simulink model "HSV"  (R2016a)
settings: Solver=VariableStepAuto  StartTime=0.0  StopTime=10.0  RelTol=1e-3
values from neighbouring files (symbols this model uses):
  arc = pi/180.    (= 0.0174532925199)    [HSV6DOF.m]    (also in Simulink_Constants.m; aerodynamics.m; initiala.m)
  bref = 24.38/2    (= 12.19)    [Simulink_Constants.m]
  CD = interp1(alX,CDX,algr,'cubic')    [aerodynamics.m]
  chi0 = -0.01    [Simulink_Constants.m]
  CL = interp1(alX,CLX,algr,'cubic')*mue    [aerodynamics.m]
  Cm = interp1(alX,CmX,algr,'cubic')    [aerodynamics.m]
  Cn = interp1(b1X,CnX,begr,'cubic')    [aerodynamics.m]
  g0 = 9.806    [Simulink_Constants.m]
  gamma0 = -0.01    [Simulink_Constants.m]
  h_theta_phi0 = [30000 55*arc 37*arc]'    [Simulink_Constants.m]
  Ix = 1572748.82    [Simulink_Constants.m]
  Ixz = 379629.026    [Simulink_Constants.m]
  Iy = 31590558.23    [Simulink_Constants.m]
  Iz = 32539630.8    [Simulink_Constants.m]
  Lref = 22.86    [Simulink_Constants.m]    (also in constants.m = 8.4088)
  m = 9300    [constants.m]
  mass_0 = 136077.7    [Simulink_Constants.m]
  mass_e = 5.4431e+04    (= 54431)    [Simulink_Constants.m]
  mass_f = 136077.7    [Simulink_Constants.m]
  phi_theta_psi_0 = [0 0 0]'    [Simulink_Constants.m]
  pqrt_0 = [0 0 0]'    [Simulink_Constants.m]
  Rearth = 6.38E6    (= 6380000)    [Simulink_Constants.m]
  rho30000m = 0.1841    [Simulink_Constants.m]
  Sref = 557.42    [Simulink_Constants.m]    (also in constants.m = 21.672)
  Ub_Vb_Qb0 = [1830 0 0]'    [Simulink_Constants.m]
  xme_0 = [0 0 0]'    [Simulink_Constants.m]
undefined symbols (not defined in the file or in its folder): Cl, Cy, Isp, magnitude, s, Thrust
libraries: aerolibutil x5, aerolibtransform2 x1, aerolibbdyn x1, aerolibconvert2 x1, aerolib6dof2 x1, aerolibanim x1, aerolibasang x1
settings Model: Creator=Bakry  LastModifiedBy=Bakry

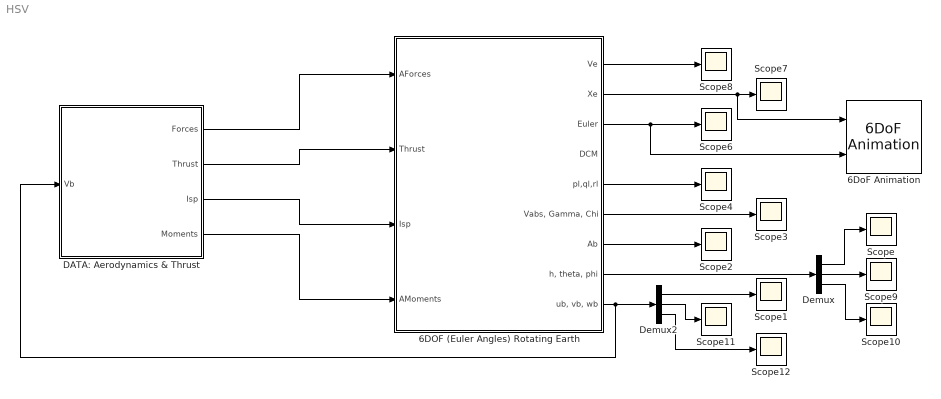
== system HSV ==
  6DOF (Euler Angles) Rotating Earth : Subsystem
  6DoF Animation : aerolibanim/6DoF Animation  u1=[0 4000 -2000 2000 -5000 -3000]  u2=0.1  u3=1.0  u4=[4000 0 -5000]  u5=Fixed position  u6=[2000 300 -3150]  u7=10  u8=on
  DATA: Aerodynamics & Thrust : Subsystem
  Demux : Demux  Outputs=3
  Demux2 : Demux  Outputs=3
  Scope{,1..4,6..12} (12 alike) : Scope
  wires:
  6DOF (Euler Angles) Rotating Earth/8("h, theta, phi") -> Demux/1
  6DOF (Euler Angles) Rotating Earth/9("ub, vb, wb") -> DATA: Aerodynamics & Thrust/1(Vb), Demux2/1
  6DOF (Euler Angles) Rotating Earth/7(Ab) -> Scope2/1
  6DOF (Euler Angles) Rotating Earth/6(" Vabs, Gamma, Chi ") -> Scope3/1
  6DOF (Euler Angles) Rotating Earth/5(pl,ql,rl) -> Scope4/1
  6DOF (Euler Angles) Rotating Earth/3(Euler) -> 6DoF Animation/2, Scope6/1
  6DOF (Euler Angles) Rotating Earth/2(Xe) -> 6DoF Animation/1, Scope7/1
  6DOF (Euler Angles) Rotating Earth/1(Ve) -> Scope8/1
  DATA: Aerodynamics & Thrust/1(Forces) -> 6DOF (Euler Angles) Rotating Earth/1(AForces)
  DATA: Aerodynamics & Thrust/2(Thrust) -> 6DOF (Euler Angles) Rotating Earth/2(Thrust)
  DATA: Aerodynamics & Thrust/3(Isp) -> 6DOF (Euler Angles) Rotating Earth/3(Isp)
  DATA: Aerodynamics & Thrust/4(Moments) -> 6DOF (Euler Angles) Rotating Earth/4(AMoments)
  Demux/1 -> Scope/1
  Demux/2 -> Scope9/1
  Demux/3 -> Scope10/1
  Demux2/2 -> Scope11/1
  Demux2/1 -> Scope1/1
  Demux2/3 -> Scope12/1

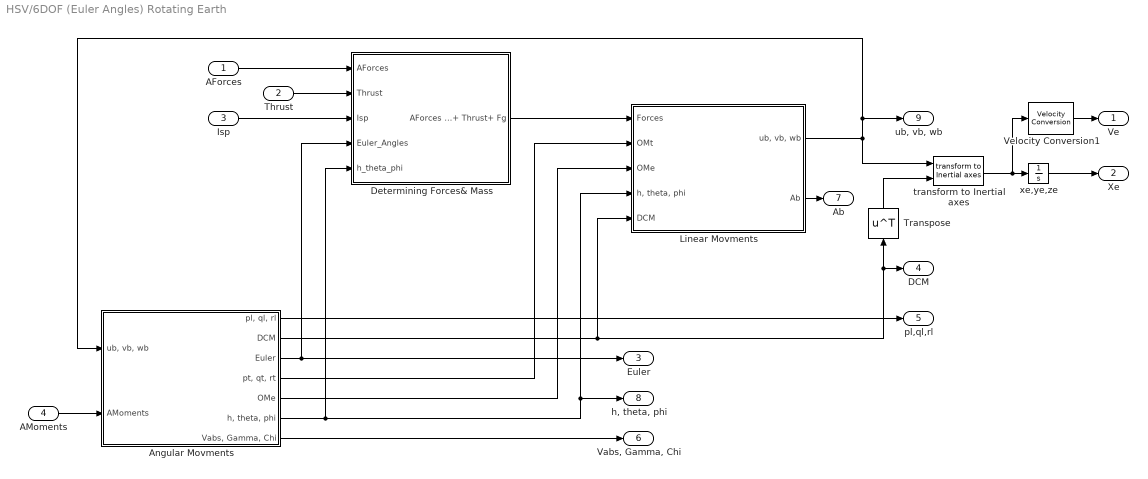
== system HSV/6DOF (Euler Angles) Rotating Earth ==
  AForces : Inport
  Thrust : Inport  Port=2
  Isp : Inport  Port=3
  AMoments : Inport  Port=4
  Angular Movments : Subsystem
  Determining Forces& Mass : Subsystem
  Linear Movments : Subsystem
  Transpose : Math  Operator=transpose  SaturateOnIntegerOverflow=on
  Velocity Conversion1 : aerolibconvert2/Velocity Conversion  IU=m/s  OU=m/s
  "transform to Inertial axes " : aerolib6dof2/6DOF (Euler Angles)/transform to Inertial axes   SystemSampleTime=-1
  xe,ye,ze : Integrator  InitialCondition=xme_0
  Ve : Outport
  Xe : Outport  Port=2
  Euler : Outport  Port=3
  DCM : Outport  Port=4
  pl,ql,rl : Outport  Port=5
  " Vabs, Gamma, Chi " : Outport  Port=6
  Ab : Outport  Port=7
  "h, theta, phi" : Outport  Port=8
  "ub, vb, wb" : Outport  Port=9
  wires:
  xe,ye,ze/1 -> Xe/1
  "transform to Inertial axes "/1 -> Velocity Conversion1/1, xe,ye,ze/1
  AForces/1 -> Determining Forces& Mass/1(AForces)
  Determining Forces& Mass/1("AForces + Thrust+ Fg ") -> Linear Movments/1(Forces)
  Transpose/1 -> "transform to Inertial axes "/2
  Thrust/1 -> Determining Forces& Mass/2(Thrust)
  Velocity Conversion1/1 -> Ve/1
  Angular Movments/2(DCM) -> DCM/1, Transpose/1, Linear Movments/5(DCM)
  Angular Movments/1("pl, ql, rl") -> pl,ql,rl/1
  Angular Movments/3(Euler) -> Euler/1, Determining Forces& Mass/4(Euler_Angles)
  Angular Movments/4("pt, qt, rt") -> Linear Movments/2(OMt)
  Angular Movments/5(OMe) -> Linear Movments/3(OMe)
  Angular Movments/6("h, theta, phi") -> "h, theta, phi"/1, Linear Movments/4("h, theta, phi"), Determining Forces& Mass/5(h_theta_phi)
  Linear Movments/1("ub, vb, wb") -> "ub, vb, wb"/1, Angular Movments/1("ub, vb, wb"), "transform to Inertial axes "/1
  Angular Movments/7(" Vabs, Gamma, Chi ") -> " Vabs, Gamma, Chi "/1
  AMoments/1 -> Angular Movments/2(AMoments)
  Isp/1 -> Determining Forces& Mass/3(Isp)
  Linear Movments/2(Ab) -> Ab/1

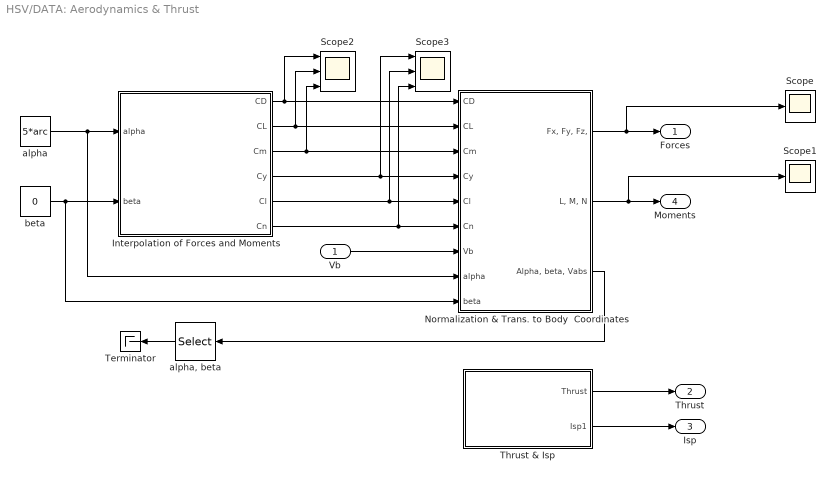
== system HSV/DATA: Aerodynamics & Thrust ==
  Vb : Inport
  Interpolation of Forces and Moments : Subsystem
  Normalization & Trans. to Body  Coordinates : Subsystem
  Scope : Scope
  Scope1 : Scope
  Scope2 : Scope  NumInputPorts=3
  Scope3 : Scope  NumInputPorts=3
  Terminator : Terminator
  Thrust & Isp : Subsystem
  alpha : Constant  Value=5*arc
  "alpha, beta" : Selector  InputPortWidth=3  IndexOptions=Index vector (dialog)  Indices=[1 2]  OutputSizes=1
  beta : Constant  Value=0
  Forces : Outport
  Thrust : Outport  Port=2
  Isp : Outport  Port=3
  Moments : Outport  Port=4
  wires:
  Interpolation of Forces and Moments/1(CD) -> Normalization & Trans. to Body  Coordinates/1(CD), Scope2/1
  Interpolation of Forces and Moments/2(CL) -> Normalization & Trans. to Body  Coordinates/2(CL), Scope2/2
  Interpolation of Forces and Moments/3(Cm) -> Normalization & Trans. to Body  Coordinates/3(Cm), Scope2/3
  Interpolation of Forces and Moments/4(Cy) -> Scope3/1, Normalization & Trans. to Body  Coordinates/4(Cy)
  Interpolation of Forces and Moments/6(Cn) -> Normalization & Trans. to Body  Coordinates/6(Cn), Scope3/3
  Vb/1 -> Normalization & Trans. to Body  Coordinates/7(Vb)
  Normalization & Trans. to Body  Coordinates/1("Fx, Fy, Fz,") -> Scope/1, Forces/1
  Normalization & Trans. to Body  Coordinates/2("L, M, N") -> Scope1/1, Moments/1
  Normalization & Trans. to Body  Coordinates/3("Alpha, beta, Vabs") -> "alpha, beta"/1
  Thrust & Isp/2(Isp1) -> Isp/1
  Thrust & Isp/1(Thrust) -> Thrust/1
  alpha/1 -> Normalization & Trans. to Body  Coordinates/8(alpha), Interpolation of Forces and Moments/1(alpha)
  beta/1 -> Interpolation of Forces and Moments/2(beta), Normalization & Trans. to Body  Coordinates/9(beta)
  "alpha, beta"/1 -> Terminator/1
  Interpolation of Forces and Moments/5(Cl) -> Scope3/2, Normalization & Trans. to Body  Coordinates/5(Cl)

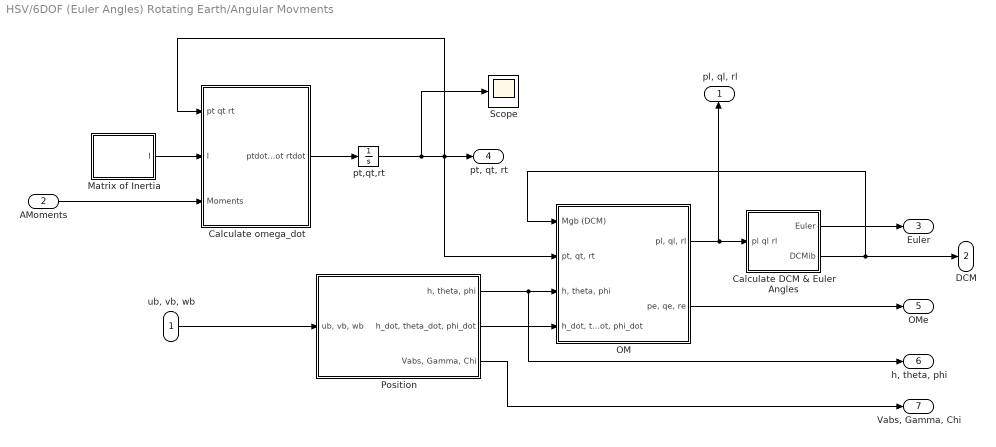
== system HSV/6DOF (Euler Angles) Rotating Earth/Angular Movments ==
  "ub, vb, wb" : Inport
  AMoments : Inport  Port=2
  Calculate DCM & Euler Angles : Subsystem
  Calculate omega_dot : Subsystem
  Matrix of Inertia : Subsystem
  OM : Subsystem
  Position : Subsystem
  Scope : Scope
  "pt,qt,rt " : Integrator  InitialCondition=pqrt_0
  "pl, ql, rl" : Outport
  DCM : Outport  Port=2
  Euler : Outport  Port=3
  "pt, qt, rt" : Outport  Port=4
  OMe : Outport  Port=5
  "h, theta, phi" : Outport  Port=6
  " Vabs, Gamma, Chi " : Outport  Port=7
  wires:
  "pt,qt,rt "/1 -> Scope/1, "pt, qt, rt"/1, OM/2("pt, qt, rt"), Calculate omega_dot/1(pt qt rt)
  Calculate omega_dot/1(ptdot qtdot rtdot) -> "pt,qt,rt "/1
  AMoments/1 -> Calculate omega_dot/3(Moments)
  Calculate DCM & Euler Angles/2(DCMib) -> OM/1(Mgb (DCM)), DCM/1
  Matrix of Inertia/1(I) -> Calculate omega_dot/2(I)
  Calculate DCM & Euler Angles/1(Euler) -> Euler/1
  "ub, vb, wb"/1 -> Position/1("ub, vb, wb")
  Position/1("h, theta, phi") -> "h, theta, phi"/1, OM/3("h, theta, phi")
  Position/2("h_dot, theta_dot, phi_dot") -> OM/4("h_dot, theta_dot, phi_dot")
  OM/1("pl, ql, rl") -> Calculate DCM & Euler Angles/1("pl ql rl "), "pl, ql, rl"/1
  OM/2("pe, qe, re") -> OMe/1
  Position/3(" Vabs, Gamma, Chi ") -> " Vabs, Gamma, Chi "/1

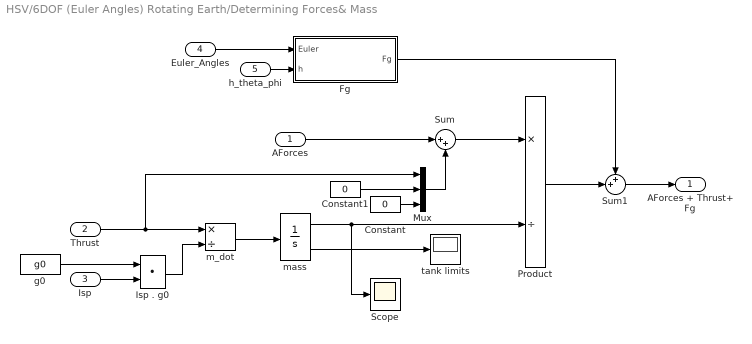
== system HSV/6DOF (Euler Angles) Rotating Earth/Determining Forces& Mass ==
  AForces : Inport
  Thrust : Inport  Port=2
  Isp : Inport  Port=3
  Euler_Angles : Inport  Port=4
  h_theta_phi : Inport  Port=5
  Constant : Constant  Value=0
  Constant1 : Constant  Value=0
  Fg : Subsystem
  Isp . g0 : DotProduct  InputSameDT=on  OutDataTypeStr=Inherit: Inherit via internal rule
  Mux : Mux  Inputs=3
  Product : Product  Inputs=*/  SaturateOnIntegerOverflow=on  OutDataTypeStr=Inherit: Same as first input
  Scope : Scope
  Sum : Sum  Inputs=|++  SaturateOnIntegerOverflow=on
  Sum1 : Sum  Inputs=++|  SaturateOnIntegerOverflow=on
  g0 : Constant  Value=g0
  m_dot : Product  Inputs=*/
  "mass  " : Integrator  InitialCondition=mass_0  LimitOutput=on  UpperSaturationLimit=mass_f  LowerSaturationLimit=mass_e  ShowSaturationPort=on
  tank limits : Display
  "AForces + Thrust+ Fg " : Outport  PortDimensions=3
  wires:
  Thrust/1 -> Mux/1, m_dot/1
  Sum/1 -> Product/1
  AForces/1 -> Sum/1
  m_dot/1 -> "mass  "/1
  "mass  "/2 -> tank limits/1
  Isp . g0/1 -> m_dot/2
  Isp/1 -> Isp . g0/2
  g0/1 -> Isp . g0/1
  "mass  "/1 -> Scope/1, Product/2
  Mux/1 -> Sum/2
  Constant/1 -> Mux/3
  Constant1/1 -> Mux/2
  Euler_Angles/1 -> Fg/1(Euler)
  h_theta_phi/1 -> Fg/2(h)
  Product/1 -> Sum1/2
  Fg/1(Fg) -> Sum1/1
  Sum1/1 -> "AForces + Thrust+ Fg "/1

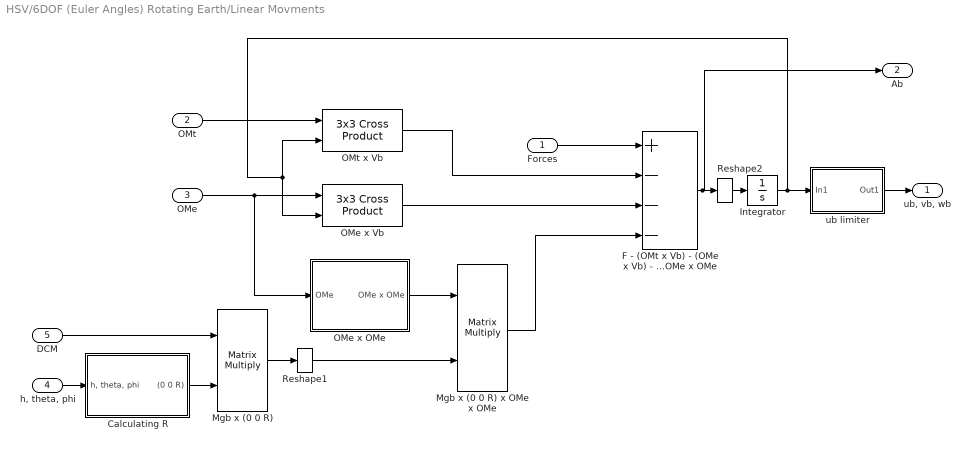
== system HSV/6DOF (Euler Angles) Rotating Earth/Linear Movments ==
  Forces : Inport
  OMt : Inport  Port=2
  OMe : Inport  Port=3
  "h, theta, phi" : Inport  Port=4
  DCM : Inport  Port=5
  Calculating R : Subsystem
  F - (OMt x Vb) - (OMe x Vb) - Mgb x (0 0 R) x OMe x OMe : Sum  Inputs=+---
  Integrator : Integrator  InitialCondition=Ub_Vb_Qb0
  Mgb x (0 0 R) : Product  Multiplication=Matrix(*)
  Mgb x (0 0 R) x OMe x OMe : Product  Multiplication=Matrix(*)
  OMe x OMe : Subsystem
  OMe x Vb : aerolibutil/3x3 Cross Product
  OMt x Vb : aerolibutil/3x3 Cross Product
  Reshape1 : Reshape  OutputDimensionality=Column vector (2-D)
  Reshape2 : Reshape  OutputDimensionality=Column vector (2-D)
  ub limiter : Subsystem
  "ub, vb, wb" : Outport
  Ab : Outport  Port=2
  wires:
  Integrator/1 -> ub limiter/1(In1), OMt x Vb/2, OMe x Vb/2
  OMt/1 -> OMt x Vb/1
  OMe/1 -> OMe x OMe/1(OMe), OMe x Vb/1
  "h, theta, phi"/1 -> Calculating R/1("h, theta, phi")
  Calculating R/1((0 0 R)) -> Mgb x (0 0 R)/2
  Mgb x (0 0 R)/1 -> Reshape1/1
  OMe x OMe/1(OMe x OMe) -> Mgb x (0 0 R) x OMe x OMe/1
  Mgb x (0 0 R) x OMe x OMe/1 -> F - (OMt x Vb) - (OMe x Vb) - Mgb x (0 0 R) x OMe x OMe/4
  OMe x Vb/1 -> F - (OMt x Vb) - (OMe x Vb) - Mgb x (0 0 R) x OMe x OMe/3
  OMt x Vb/1 -> F - (OMt x Vb) - (OMe x Vb) - Mgb x (0 0 R) x OMe x OMe/2
  Forces/1 -> F - (OMt x Vb) - (OMe x Vb) - Mgb x (0 0 R) x OMe x OMe/1
  F - (OMt x Vb) - (OMe x Vb) - Mgb x (0 0 R) x OMe x OMe/1 -> Ab/1, Reshape2/1
  ub limiter/1(Out1) -> "ub, vb, wb"/1
  DCM/1 -> Mgb x (0 0 R)/1
  Reshape1/1 -> Mgb x (0 0 R) x OMe x OMe/2
  Reshape2/1 -> Integrator/1

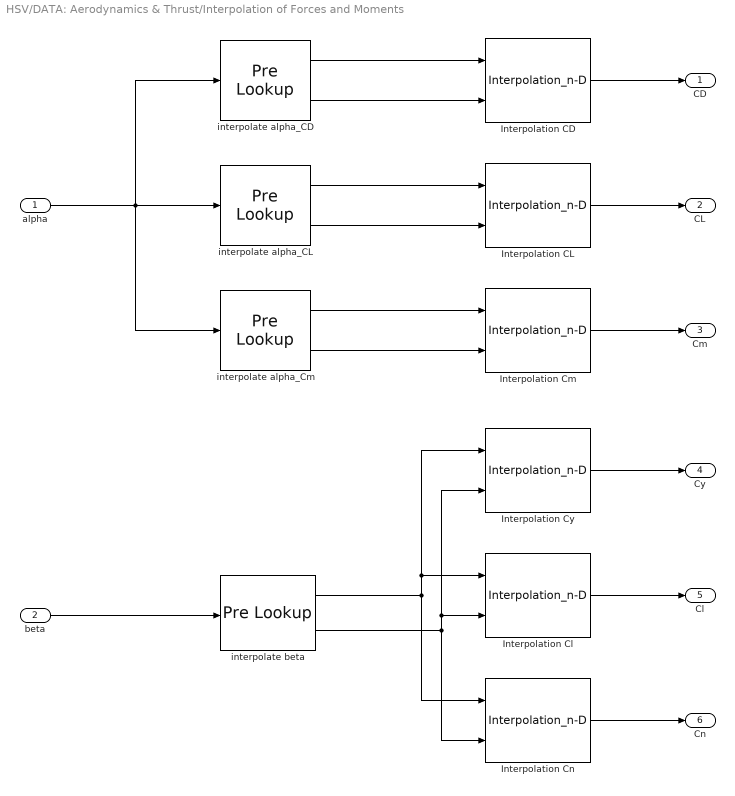
== system HSV/DATA: Aerodynamics & Thrust/Interpolation of Forces and Moments ==
  alpha : Inport
  beta : Inport  Port=2
  Interpolation CD : Interpolation_n-D  NumberOfTableDimensions=1  Table=CD(:,2)  InternalRulePriority=Speed
      settings: InputPortMap=u0,u1
  Interpolation CL : Interpolation_n-D  NumberOfTableDimensions=1  Table=CL(:,2)  InternalRulePriority=Speed
      settings: InputPortMap=u0,u1
  Interpolation Cl : Interpolation_n-D  NumberOfTableDimensions=1  Table=Cl(:,2)  InternalRulePriority=Speed
      settings: InputPortMap=u0,u1
  Interpolation Cm : Interpolation_n-D  NumberOfTableDimensions=1  Table=Cm(:,2)  InternalRulePriority=Speed
      settings: InputPortMap=u0,u1
  Interpolation Cn : Interpolation_n-D  NumberOfTableDimensions=1  Table=Cn(:,2)  InternalRulePriority=Speed
      settings: InputPortMap=u0,u1
  Interpolation Cy : Interpolation_n-D  NumberOfTableDimensions=1  Table=Cy(:,2)  InternalRulePriority=Speed
      settings: InputPortMap=u0,u1
  interpolate alpha_CD : PreLookup  BreakpointsData=alpha_CD  ExtrapMethod=Linear
  interpolate alpha_CL : PreLookup  BreakpointsData=alpha_CL  ExtrapMethod=Linear
  interpolate alpha_Cm : PreLookup  BreakpointsData=alpha_Cm  ExtrapMethod=Linear
  interpolate beta : PreLookup  BreakpointsData=beta_Cy  ExtrapMethod=Linear
  CD : Outport
  CL : Outport  Port=2
  Cm : Outport  Port=3
  Cy : Outport  Port=4
  Cl : Outport  Port=5
  Cn : Outport  Port=6
  wires:
  Interpolation CD/1 -> CD/1
  Interpolation Cl/1 -> Cl/1
  Interpolation Cn/1 -> Cn/1
  Interpolation Cy/1 -> Cy/1
  interpolate beta/2 -> Interpolation Cl/2, Interpolation Cy/2, Interpolation Cn/2
  interpolate beta/1 -> Interpolation Cl/1, Interpolation Cy/1, Interpolation Cn/1
  beta/1 -> interpolate beta/1
  Interpolation Cm/1 -> Cm/1
  Interpolation CL/1 -> CL/1
  alpha/1 -> interpolate alpha_Cm/1, interpolate alpha_CL/1, interpolate alpha_CD/1
  interpolate alpha_CD/1 -> Interpolation CD/1
  interpolate alpha_CD/2 -> Interpolation CD/2
  interpolate alpha_CL/1 -> Interpolation CL/1
  interpolate alpha_CL/2 -> Interpolation CL/2
  interpolate alpha_Cm/1 -> Interpolation Cm/1
  interpolate alpha_Cm/2 -> Interpolation Cm/2

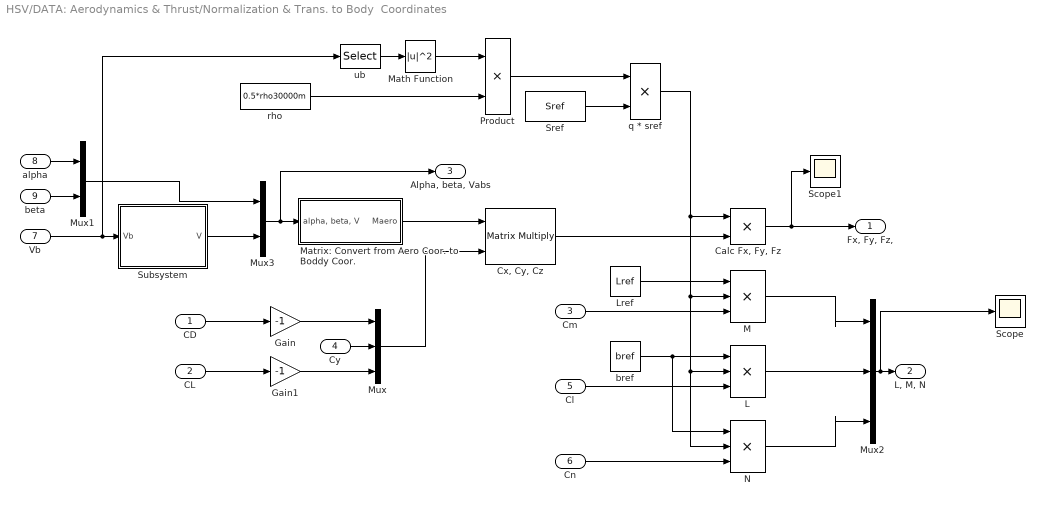
== system HSV/DATA: Aerodynamics & Thrust/Normalization & Trans. to Body  Coordinates ==
  CD : Inport
  CL : Inport  Port=2
  Cm : Inport  Port=3
  Cy : Inport  Port=4
  Cl : Inport  Port=5
  Cn : Inport  Port=6
  Vb : Inport  Port=7
  alpha : Inport  Port=8
  beta : Inport  Port=9
  "Calc Fx, Fy, Fz" : Product
  "Cx, Cy, Cz" : Product  Multiplication=Matrix(*)
  Gain : Gain  Gain=-1
  Gain1 : Gain  Gain=-1
  L : Product  Inputs=3
  Lref : Constant  Value=Lref
  M : Product  Inputs=3
  Math Function : Math  Operator=magnitude^2  SaturateOnIntegerOverflow=on
  Matrix: Convert from Aero Coor. to Boddy Coor. : Subsystem
  Mux : Mux  Inputs=3
  Mux1 : Mux  Inputs=2
  Mux2 : Mux  Inputs=3
  Mux3 : Mux  Inputs=2
  N : Product  Inputs=3
  Product : Product
  Scope : Scope
  Scope1 : Scope
  Sref : Constant  Value=Sref
  Subsystem : Subsystem
  bref : Constant  Value=bref
  q * sref : Product
  rho : Constant  Value=0.5*rho30000m
  ub : Selector  InputPortWidth=3  IndexOptions=Index vector (dialog)  Indices=[1]  OutputSizes=1
  "Fx, Fy, Fz," : Outport
  "L, M, N" : Outport  Port=2
  "Alpha, beta, Vabs" : Outport  Port=3
  wires:
  CD/1 -> Gain/1
  CL/1 -> Gain1/1
  Gain/1 -> Mux/1
  Cy/1 -> Mux/2
  Gain1/1 -> Mux/3
  Matrix: Convert from Aero Coor. to Boddy Coor./1(Maero) -> "Cx, Cy, Cz"/1
  Mux/1 -> "Cx, Cy, Cz"/2
  Product/1 -> q * sref/1
  Sref/1 -> q * sref/2
  q * sref/1 -> N/2, L/2, M/2, "Calc Fx, Fy, Fz"/1
  "Cx, Cy, Cz"/1 -> "Calc Fx, Fy, Fz"/2
  Cm/1 -> M/3
  Lref/1 -> M/1
  Cl/1 -> L/3
  bref/1 -> L/1, N/1
  Cn/1 -> N/3
  Mux2/1 -> Scope/1, "L, M, N"/1
  L/1 -> Mux2/2
  M/1 -> Mux2/1
  N/1 -> Mux2/3
  "Calc Fx, Fy, Fz"/1 -> Scope1/1, "Fx, Fy, Fz,"/1
  Vb/1 -> ub/1, Subsystem/1(Vb)
  alpha/1 -> Mux1/1
  beta/1 -> Mux1/2
  Mux1/1 -> Mux3/1
  Subsystem/1(V) -> Mux3/2
  Mux3/1 -> "Alpha, beta, Vabs"/1, Matrix: Convert from Aero Coor. to Boddy Coor./1("alpha, beta, V")
  rho/1 -> Product/2
  ub/1 -> Math Function/1
  Math Function/1 -> Product/1

== system HSV/DATA: Aerodynamics & Thrust/Thrust & Isp ==
  Given Isp : Constant  Value=Isp
  Given Thrust : Constant  Value=Thrust
  Thrust : Outport
  Isp1 : Outport  Port=2
  wires:
  Given Isp/1 -> Isp1/1
  Given Thrust/1 -> Thrust/1

== system HSV/6DOF (Euler Angles) Rotating Earth/Angular Movments/Calculate DCM & Euler Angles ==
  "pl ql rl " : Inport
  Euler Limits : Subsystem
  Rotation Angles to Direction Cosine Matrix : aerolibtransform2/Rotation Angles to Direction Cosine Matrix  rotationOrder=ZYX
  Selector : Selector  InputPortWidth=3  IndexOptions=Index vector (dialog)  Indices=[3 2 1]  OutputSizes=1
  phi theta psi : Integrator  InitialCondition=phi_theta_psi_0
  phidot thetadot psidot : Subsystem
  Euler : Outport
  DCMib : Outport  Port=2
  wires:
  Rotation Angles to Direction Cosine Matrix/1 -> DCMib/1
  "pl ql rl "/1 -> phidot thetadot psidot/1(p q r)
  phidot thetadot psidot/1(phidot thetadot psi) -> phi theta psi/1
  phi theta psi/1 -> phidot thetadot psidot/2(phi theta psi), Euler Limits/1("phi, theta, psi"), Selector/1
  Selector/1 -> Rotation Angles to Direction Cosine Matrix/1
  Euler Limits/1("Limited phi, theta, psi") -> Euler/1

== system HSV/6DOF (Euler Angles) Rotating Earth/Angular Movments/Calculate omega_dot ==
  pt qt rt : Inport
  I : Inport  Port=2
  Moments : Inport  Port=3
  Product2 : Product  Inputs=*/  Multiplication=Matrix(*)  SaturateOnIntegerOverflow=on  OutDataTypeStr=Inherit: Same as first input
  Reshape : Reshape
  Reshape1 : Reshape  OutputDimensionality=Row vector (2-D)
  Subsystem1 : Subsystem
  Sum2 : Sum  Inputs=+-  SaturateOnIntegerOverflow=on
  wx(Iw) : aerolibutil/3x3 Cross Product
  ptdot qtdot rtdot : Outport
  wires:
  Reshape1/1 -> Product2/1
  Subsystem1/1(I * w) -> wx(Iw)/2
  wx(Iw)/1 -> Sum2/2
  Moments/1 -> Sum2/1
  Sum2/1 -> Reshape1/1
  Product2/1 -> Reshape/1
  pt qt rt/1 -> Subsystem1/1(pt qt rt), wx(Iw)/1
  I/1 -> Subsystem1/2(Inertia), Product2/2
  Reshape/1 -> ptdot qtdot rtdot/1

== system HSV/6DOF (Euler Angles) Rotating Earth/Angular Movments/Matrix of Inertia ==
  note: T(1,1) = 4932.; T(1,2) = 0.;     T(1,3) =-3155.;
      | T(2,1) = 0.;    T(2,2) = 60338.; T(2,3) = 0.;
      | T(3,1) =-3155.; T(3,2) = 0.;     T(3,3) = 62561.;
  Ix : Constant  Value=Ix
  Ixz : Constant  Value=Ixz
  Ixz1 : Constant  Value=0
  Ixz2 : Constant  Value=0
  Iy : Constant  Value=Iy
  Iz : Constant  Value=Iz
  Symmetric Inertia Tensor : aerolibbdyn/Symmetric Inertia Tensor
  I : Outport
  wires:
  Symmetric Inertia Tensor/1 -> I/1
  Ix/1 -> Symmetric Inertia Tensor/1
  Iy/1 -> Symmetric Inertia Tensor/4
  Iz/1 -> Symmetric Inertia Tensor/6
  Ixz/1 -> Symmetric Inertia Tensor/3
  Ixz1/1 -> Symmetric Inertia Tensor/2
  Ixz2/1 -> Symmetric Inertia Tensor/5

== system HSV/6DOF (Euler Angles) Rotating Earth/Angular Movments/OM ==
  Mgb (DCM) : Inport
  "pt, qt, rt" : Inport  Port=2
  "h, theta, phi" : Inport  Port=3
  "h_dot, theta_dot, phi_dot" : Inport  Port=4
  "Calculating pe, qe, re" : Subsystem
  "Calculating pl, ql, rl" : Subsystem
  "p, q, r" : Subsystem
  "pl, ql, rl" : Outport
  "pe, qe, re" : Outport  Port=2
  wires:
  "Calculating pe, qe, re"/1("pe, qe, re") -> "pe, qe, re"/1, "Calculating pl, ql, rl"/2("pe, qe, re")
  Mgb (DCM)/1 -> "Calculating pe, qe, re"/1(Mgb = DCM), "p, q, r"/1(Mgb = DCM)
  "pt, qt, rt"/1 -> "Calculating pl, ql, rl"/1("pt, qt, rt")
  "h, theta, phi"/1 -> "p, q, r"/2("h, theta, phi"), "Calculating pe, qe, re"/2("h, theta, phi")
  "p, q, r"/1("p, q, r") -> "Calculating pl, ql, rl"/3("p, q, r")
  "h_dot, theta_dot, phi_dot"/1 -> "p, q, r"/3("h_dot, theta_dot, phi_dot")
  "Calculating pl, ql, rl"/1("pl, ql, rl") -> "pl, ql, rl"/1

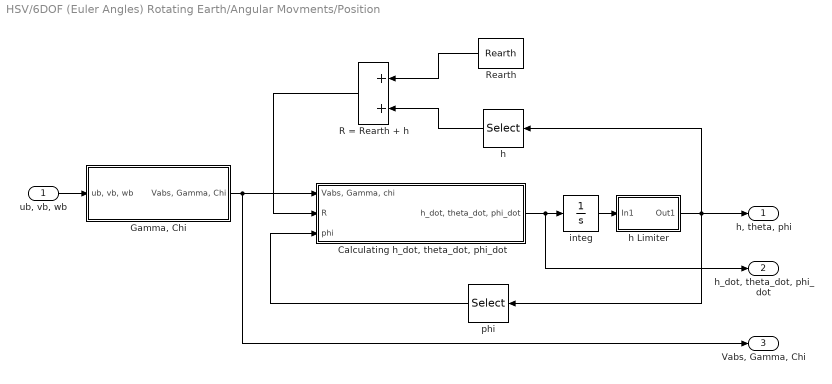
== system HSV/6DOF (Euler Angles) Rotating Earth/Angular Movments/Position ==
  "ub, vb, wb" : Inport
  "Calculating h_dot, theta_dot, phi_dot" : Subsystem
  "Gamma, Chi" : Subsystem
  R = Rearth + h : Sum
  Rearth : Constant  Value=Rearth
  h : Selector  InputPortWidth=3  IndexOptions=Index vector (dialog)  Indices=[1]  OutputSizes=1
  h Limiter : Subsystem
  "integ " : Integrator  InitialCondition=h_theta_phi0
  phi : Selector  InputPortWidth=3  IndexOptions=Index vector (dialog)  Indices=[3]  OutputSizes=1
  "h, theta, phi" : Outport
  "h_dot, theta_dot, phi_dot" : Outport  Port=2
  " Vabs, Gamma, Chi " : Outport  Port=3
  wires:
  "ub, vb, wb"/1 -> "Gamma, Chi"/1("ub, vb, wb")
  "Calculating h_dot, theta_dot, phi_dot"/1("h_dot, theta_dot, phi_dot") -> "integ "/1, "h_dot, theta_dot, phi_dot"/1
  "integ "/1 -> h Limiter/1(In1)
  phi/1 -> "Calculating h_dot, theta_dot, phi_dot"/3(phi)
  "Gamma, Chi"/1(" Vabs, Gamma, Chi ") -> " Vabs, Gamma, Chi "/1, "Calculating h_dot, theta_dot, phi_dot"/1("Vabs, Gamma, chi")
  h/1 -> R = Rearth + h/2
  Rearth/1 -> R = Rearth + h/1
  R = Rearth + h/1 -> "Calculating h_dot, theta_dot, phi_dot"/2(R)
  h Limiter/1(Out1) -> phi/1, h/1, "h, theta, phi"/1

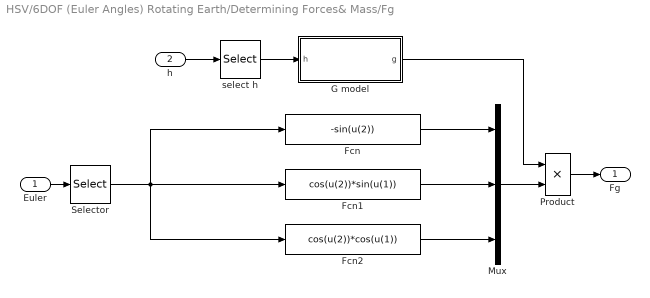
== system HSV/6DOF (Euler Angles) Rotating Earth/Determining Forces& Mass/Fg ==
  Euler : Inport
  h : Inport  Port=2
  Fcn : Fcn  Expr=-sin(u(2))
  Fcn1 : Fcn  Expr=cos(u(2))*sin(u(1))
  Fcn2 : Fcn  Expr=cos(u(2))*cos(u(1))
  G model : Subsystem
  Mux : Mux  Inputs=3
  Product : Product
  Selector : Selector  InputPortWidth=3  IndexOptions=Index vector (dialog)  Indices=[1 2]  OutputSizes=1
  select h : Selector  InputPortWidth=3  IndexOptions=Index vector (dialog)  Indices=[1]  OutputSizes=1
  Fg : Outport
  wires:
  Fcn1/1 -> Mux/2
  Fcn/1 -> Mux/1
  Fcn2/1 -> Mux/3
  Mux/1 -> Product/2
  Euler/1 -> Selector/1
  Selector/1 -> Fcn/1, Fcn2/1, Fcn1/1
  h/1 -> select h/1
  select h/1 -> G model/1(h)
  Product/1 -> Fg/1
  G model/1(g) -> Product/1

== system HSV/6DOF (Euler Angles) Rotating Earth/Linear Movments/Calculating R ==
  "h, theta, phi" : Inport
  Constant : Constant  Value=0
  Constant1 : Constant  Value=0
  Mux : Mux  Inputs=3
  R = Rearth + h : Sum
  Rearth : Constant  Value=Rearth
  h : Selector  InputPortWidth=3  IndexOptions=Index vector (dialog)  Indices=[1]  OutputSizes=1
  (0 0 R) : Outport
  wires:
  h/1 -> R = Rearth + h/1
  "h, theta, phi"/1 -> h/1
  Rearth/1 -> R = Rearth + h/2
  Mux/1 -> (0 0 R)/1
  R = Rearth + h/1 -> Mux/3
  Constant1/1 -> Mux/2
  Constant/1 -> Mux/1

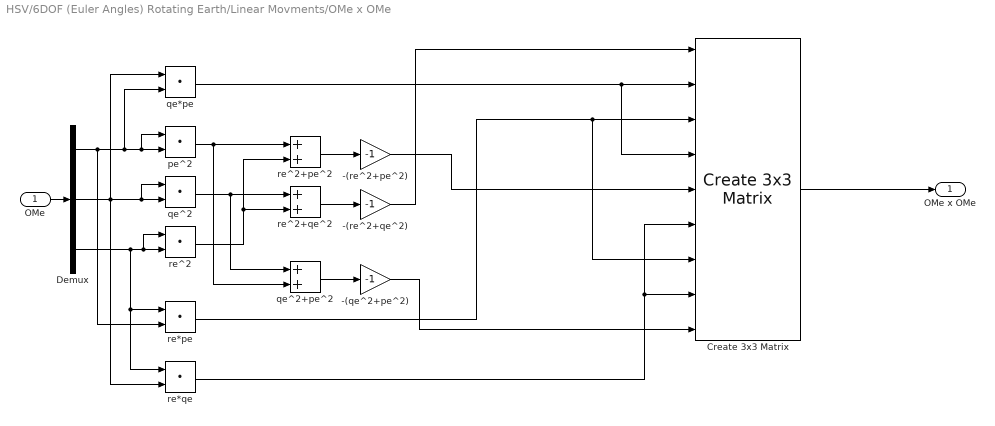
== system HSV/6DOF (Euler Angles) Rotating Earth/Linear Movments/OMe x OMe ==
  OMe : Inport
  -(qe^2+pe^2) : Gain  Gain=-1
  -(re^2+pe^2) : Gain  Gain=-1
  -(re^2+qe^2) : Gain  Gain=-1
  Create 3x3 Matrix : aerolibutil/Create 3x3 Matrix
  Demux : Demux  Outputs=3
  pe^2 : DotProduct  InputSameDT=on  OutDataTypeStr=Inherit: Inherit via internal rule
  qe*pe : DotProduct  InputSameDT=on  OutDataTypeStr=Inherit: Inherit via internal rule
  qe^2 : DotProduct  InputSameDT=on  OutDataTypeStr=Inherit: Inherit via internal rule
  qe^2+pe^2 : Sum
  re*pe : DotProduct  InputSameDT=on  OutDataTypeStr=Inherit: Inherit via internal rule
  re*qe : DotProduct  InputSameDT=on  OutDataTypeStr=Inherit: Inherit via internal rule
  re^2 : DotProduct  InputSameDT=on  OutDataTypeStr=Inherit: Inherit via internal rule
  re^2+pe^2 : Sum
  re^2+qe^2 : Sum
  OMe x OMe : Outport
  wires:
  Create 3x3 Matrix/1 -> OMe x OMe/1
  OMe/1 -> Demux/1
  Demux/1 -> re*pe/2, qe*pe/2, pe^2/1, pe^2/2
  Demux/2 -> re*qe/2, qe*pe/1, qe^2/2, qe^2/1
  Demux/3 -> re*qe/1, re*pe/1, re^2/1, re^2/2
  re^2+qe^2/1 -> -(re^2+qe^2)/1
  -(re^2+qe^2)/1 -> Create 3x3 Matrix/1
  re^2/1 -> re^2+pe^2/2, re^2+qe^2/2
  re^2+pe^2/1 -> -(re^2+pe^2)/1
  -(re^2+pe^2)/1 -> Create 3x3 Matrix/5
  pe^2/1 -> re^2+pe^2/1, qe^2+pe^2/2
  qe^2+pe^2/1 -> -(qe^2+pe^2)/1
  qe^2/1 -> re^2+qe^2/1, qe^2+pe^2/1
  -(qe^2+pe^2)/1 -> Create 3x3 Matrix/9
  qe*pe/1 -> Create 3x3 Matrix/4, Create 3x3 Matrix/2
  re*pe/1 -> Create 3x3 Matrix/7, Create 3x3 Matrix/3
  re*qe/1 -> Create 3x3 Matrix/8, Create 3x3 Matrix/6

== system HSV/6DOF (Euler Angles) Rotating Earth/Linear Movments/ub limiter ==
  In1 : Inport
  Demux : Demux  Outputs=3
  Gain : Gain  Gain=-1
  Mux : Mux  Inputs=3
  Saturation1 : Saturate  UpperLimit=2000  LowerLimit=1850
  Saturation2 : Saturate  UpperLimit=1  LowerLimit=-1
  Saturation3 : Saturate
  Out1 : Outport
  wires:
  In1/1 -> Demux/1
  Mux/1 -> Out1/1
  Demux/2 -> Saturation3/1
  Demux/3 -> Saturation2/1
  Demux/1 -> Saturation1/1
  Saturation2/1 -> Gain/1
  Saturation3/1 -> Mux/2
  Saturation1/1 -> Mux/1
  Gain/1 -> Mux/3

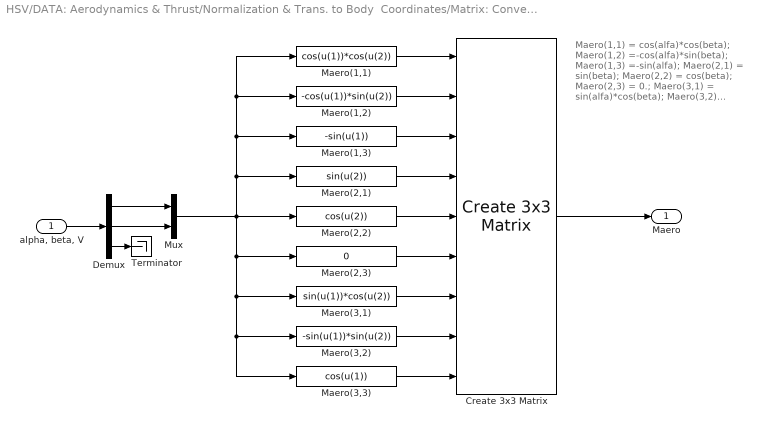
== system HSV/DATA: Aerodynamics & Thrust/Normalization & Trans. to Body  Coordinates/Matrix: Convert from Aero Coor. to Boddy Coor. ==
  note: Maero(1,1) = cos(alfa)*cos(beta);
      | Maero(1,2) =-cos(alfa)*sin(beta);
      | Maero(1,3) =-sin(alfa);
      | Maero(2,1) = sin(beta);
      | Maero(2,2) = cos(beta);
      | Maero(2,3) = 0.;
      | Maero(3,1) = sin(alfa)*cos(beta);
      | Maero(3,2) =-sin(alfa)*sin(beta);
      | Maero(3,3) = cos(alfa);
  "alpha, beta, V" : Inport
  Create 3x3 Matrix : aerolibutil/Create 3x3 Matrix
  Demux : Demux  Outputs=3
  "Maero(1,1) " : Fcn  Expr=cos(u(1))*cos(u(2))
  Maero(1,2) : Fcn  Expr=-cos(u(1))*sin(u(2))
  "Maero(1,3) " : Fcn  Expr=-sin(u(1))
  Maero(2,1) : Fcn  Expr=sin(u(2))
  Maero(2,2) : Fcn  Expr=cos(u(2))
  Maero(2,3) : Fcn  Expr=0
  Maero(3,1) : Fcn  Expr=sin(u(1))*cos(u(2))
  Maero(3,2) : Fcn  Expr=-sin(u(1))*sin(u(2))
  Maero(3,3) : Fcn  Expr=cos(u(1))
  Mux : Mux  Inputs=2
  Terminator : Terminator
  Maero : Outport
  wires:
  "alpha, beta, V"/1 -> Demux/1
  Demux/1 -> Mux/1
  Demux/3 -> Terminator/1
  Demux/2 -> Mux/2
  Mux/1 -> "Maero(1,3) "/1, Maero(1,2)/1, "Maero(1,1) "/1, Maero(2,1)/1, Maero(3,3)/1, Maero(3,2)/1, Maero(3,1)/1, Maero(2,3)/1, Maero(2,2)/1
  "Maero(1,1) "/1 -> Create 3x3 Matrix/1
  Maero(1,2)/1 -> Create 3x3 Matrix/2
  "Maero(1,3) "/1 -> Create 3x3 Matrix/3
  Maero(2,1)/1 -> Create 3x3 Matrix/4
  Maero(2,2)/1 -> Create 3x3 Matrix/5
  Maero(2,3)/1 -> Create 3x3 Matrix/6
  Maero(3,1)/1 -> Create 3x3 Matrix/7
  Maero(3,2)/1 -> Create 3x3 Matrix/8
  Maero(3,3)/1 -> Create 3x3 Matrix/9
  Create 3x3 Matrix/1 -> Maero/1

== system HSV/DATA: Aerodynamics & Thrust/Normalization & Trans. to Body  Coordinates/Subsystem ==
  Vb : Inport
  "Incidence, Sideslip, & Airspeed" : aerolibasang/Incidence, Sideslip, & Airspeed
  Saturation : Saturate  UpperLimit=21*arc  LowerLimit=-3*arc
  Saturation1 : Saturate  UpperLimit=0  LowerLimit=0
  Terminator : Terminator
  Terminator1 : Terminator
  V : Outport
  wires:
  "Incidence, Sideslip, & Airspeed"/2 -> Saturation1/1
  Saturation1/1 -> Terminator1/1
  "Incidence, Sideslip, & Airspeed"/3 -> V/1
  Vb/1 -> "Incidence, Sideslip, & Airspeed"/1
  "Incidence, Sideslip, & Airspeed"/1 -> Saturation/1
  Saturation/1 -> Terminator/1

== system HSV/6DOF (Euler Angles) Rotating Earth/Angular Movments/Calculate DCM & Euler Angles/Euler Limits ==
  "phi, theta, psi" : Inport
  Demux : Demux  Outputs=3
  Mux : Mux  Inputs=3
  phi : Saturate  UpperLimit=45*arc  LowerLimit=-45*arc
  psi : Saturate  UpperLimit=180*arc  LowerLimit=-180*arc
  theta : Saturate  UpperLimit=89*arc  LowerLimit=-89*arc
  "Limited phi, theta, psi" : Outport
  wires:
  Mux/1 -> "Limited phi, theta, psi"/1
  "phi, theta, psi"/1 -> Demux/1
  Demux/1 -> phi/1
  phi/1 -> Mux/1
  Demux/3 -> psi/1
  psi/1 -> Mux/3
  theta/1 -> Mux/2
  Demux/2 -> theta/1

== system HSV/6DOF (Euler Angles) Rotating Earth/Angular Movments/Calculate DCM & Euler Angles/phidot thetadot psidot ==
  p q r : Inport
  phi theta psi : Inport  Port=2
  Mux1 : Mux  Inputs=[3 3 3]
  Mux2 : Mux  Inputs=3
  phidot : Fcn  Expr=u[1]+(u[2]*u[4]+u[3]*u[7])*(u[5]/u[8])
  psidot : Fcn  Expr=(u[2]*u[4]+u[3]*u[7])/u[8]
  sincos : Trigonometry  Operator=sincos
  thetadot : Fcn  Expr=u[2]*u[7]-u[3]*u[4]
  phidot thetadot psi : Outport  InitialOutput=0
  wires:
  Mux1/1 -> psidot/1, phidot/1, thetadot/1
  p q r/1 -> Mux1/1
  phi theta psi/1 -> sincos/1
  psidot/1 -> Mux2/3
  thetadot/1 -> Mux2/2
  phidot/1 -> Mux2/1
  Mux2/1 -> phidot thetadot psi/1
  sincos/1 -> Mux1/2
  sincos/2 -> Mux1/3

== system HSV/6DOF (Euler Angles) Rotating Earth/Angular Movments/Calculate omega_dot/Subsystem1 ==
  pt qt rt : Inport
  Inertia : Inport  Port=2
  Product : Product  Multiplication=Matrix(*)  SaturateOnIntegerOverflow=on  InputSameDT=on  OutDataTypeStr=Inherit: Same as first input
  Reshape1 : Reshape  OutputDimensionality=Column vector (2-D)
  Reshape2 : Reshape
  I * w : Outport
  wires:
  Reshape2/1 -> I * w/1
  Reshape1/1 -> Product/2
  pt qt rt/1 -> Reshape1/1
  Inertia/1 -> Product/1
  Product/1 -> Reshape2/1

== system HSV/6DOF (Euler Angles) Rotating Earth/Angular Movments/OM/Calculating pe, qe, re ==
  Mgb = DCM : Inport
  "h, theta, phi" : Inport  Port=2
  Mgb * Om_dash|g : Product  Multiplication=Matrix(*)
  Om_dash|g : Subsystem
  phi1 : Selector  InputPortWidth=3  IndexOptions=Index vector (dialog)  Indices=[3]  OutputSizes=1
  "pe, qe, re" : Outport
  wires:
  Mgb = DCM/1 -> Mgb * Om_dash|g/1
  Mgb * Om_dash|g/1 -> "pe, qe, re"/1
  "h, theta, phi"/1 -> phi1/1
  Om_dash|g/1(Om_dash|b) -> Mgb * Om_dash|g/2
  phi1/1 -> Om_dash|g/1(phi)

== system HSV/6DOF (Euler Angles) Rotating Earth/Angular Movments/OM/Calculating pl, ql, rl ==
  "pt, qt, rt" : Inport
  "pe, qe, re" : Inport  Port=2
  "p, q, r" : Inport  Port=3
  Ome + Om : Sum
  Oml - (Ome + Om) : Sum  Inputs=+-
  "pl, ql, rl" : Outport
  wires:
  "pe, qe, re"/1 -> Ome + Om/1
  "p, q, r"/1 -> Ome + Om/2
  Ome + Om/1 -> Oml - (Ome + Om)/2
  "pt, qt, rt"/1 -> Oml - (Ome + Om)/1
  Oml - (Ome + Om)/1 -> "pl, ql, rl"/1

== system HSV/6DOF (Euler Angles) Rotating Earth/Angular Movments/OM/p, q, r ==
  Mgb = DCM : Inport
  "h, theta, phi" : Inport  Port=2
  "h_dot, theta_dot, phi_dot" : Inport  Port=3
  Mgb * Om|g : Product  Multiplication=Matrix(*)
  Mux : Mux  Inputs=2
  Om|g : Subsystem
  phi : Selector  InputPortWidth=3  IndexOptions=Index vector (dialog)  Indices=[3]  OutputSizes=1
  "theta_dot, phi_dot" : Selector  InputPortWidth=3  IndexOptions=Index vector (dialog)  Indices=[2 3]  OutputSizes=1
  "p, q, r" : Outport
  wires:
  Om|g/1(Om_dash|b) -> Mgb * Om|g/2
  Mgb * Om|g/1 -> "p, q, r"/1
  Mgb = DCM/1 -> Mgb * Om|g/1
  "h_dot, theta_dot, phi_dot"/1 -> "theta_dot, phi_dot"/1
  "h, theta, phi"/1 -> phi/1
  Mux/1 -> Om|g/1("theta_dot, phi_dot, phi")
  phi/1 -> Mux/1
  "theta_dot, phi_dot"/1 -> Mux/2

== system HSV/6DOF (Euler Angles) Rotating Earth/Angular Movments/Position/Calculating h_dot, theta_dot, phi_dot ==
  note: u1 = V, u2 = Gamma, u3 = chi, u4 = R, u5 = phi
  "Vabs, Gamma, chi" : Inport
  R : Inport  Port=2
  phi : Inport  Port=3
  Mux : Mux  Inputs=3
  Mux1 : Mux  Inputs=3
  h_dot : Fcn  Expr=u(1)*sin(u(2))
  phi_dot : Fcn  Expr=u(1)*cos(u(2))*cos(u(3))/u(4)
  theta_dot : Fcn  Expr=u(1)*cos(u(2))*sin(u(3))/(u(4)*cos(u(5)))
  "h_dot, theta_dot, phi_dot" : Outport
  wires:
  phi_dot/1 -> Mux/3
  Mux/1 -> "h_dot, theta_dot, phi_dot"/1
  theta_dot/1 -> Mux/2
  "Vabs, Gamma, chi"/1 -> Mux1/1
  h_dot/1 -> Mux/1
  R/1 -> Mux1/2
  phi/1 -> Mux1/3
  Mux1/1 -> phi_dot/1, h_dot/1, theta_dot/1

== system HSV/6DOF (Euler Angles) Rotating Earth/Angular Movments/Position/Gamma, Chi ==
  note: u1 = u, u2 = v, u3 = w
  "ub, vb, wb" : Inport
  Chi : Fcn  Expr=atan(u(2)/u(1))
  Chi 0 : Constant  Value=chi0
  Gamma : Fcn  Expr=-asin(u(3)/u(4))
  Gamma 0 : Constant  Value=gamma0
  Mux : Mux  Inputs=2
  Mux1 : Mux  Inputs=3
  Subtract : Sum
  Subtract1 : Sum
  Vabs : Fcn  Expr=sqrt(u(1)*u(1)+u(2)*u(2)+u(3)*u(3))
  " Vabs, Gamma, Chi " : Outport
  wires:
  "ub, vb, wb"/1 -> Mux/1, Vabs/1
  Vabs/1 -> Mux1/1, Mux/2
  Mux/1 -> Chi/1, Gamma/1
  Chi/1 -> Subtract1/1
  Gamma/1 -> Subtract/2
  Mux1/1 -> " Vabs, Gamma, Chi "/1
  Gamma 0/1 -> Subtract/1
  Chi 0/1 -> Subtract1/2
  Subtract/1 -> Mux1/2
  Subtract1/1 -> Mux1/3

== system HSV/6DOF (Euler Angles) Rotating Earth/Angular Movments/Position/h Limiter ==
  In1 : Inport
  Demux : Demux  Outputs=3
  Mux : Mux  Inputs=3
  Saturation : Saturate  UpperLimit=30100  LowerLimit=29900
  Saturation1 : Saturate  UpperLimit=180*arc  LowerLimit=-180*arc
  Saturation2 : Saturate  UpperLimit=89*arc  LowerLimit=-89*arc
  Out1 : Outport
  wires:
  Mux/1 -> Out1/1
  In1/1 -> Demux/1
  Demux/2 -> Saturation1/1
  Demux/3 -> Saturation2/1
  Saturation/1 -> Mux/1
  Demux/1 -> Saturation/1
  Saturation1/1 -> Mux/2
  Saturation2/1 -> Mux/3

== system HSV/6DOF (Euler Angles) Rotating Earth/Determining Forces& Mass/Fg/G model ==
  h : Inport
  Fcn : Fcn  Expr=g0*(Rearth/(Rearth+u(1)))^2
  g : Outport
  wires:
  h/1 -> Fcn/1
  Fcn/1 -> g/1

== system HSV/6DOF (Euler Angles) Rotating Earth/Angular Movments/OM/Calculating pe, qe, re/Om_dash|g ==
  phi : Inport
  Constant : Constant  Value=0
  Fcn : Fcn  Expr=cos(u)
  Fcn1 : Fcn  Expr=-sin(u)
  Mux : Mux  Inputs=3
  Om_dash|b : Outport
  wires:
  phi/1 -> Fcn1/1, Fcn/1
  Constant/1 -> Mux/2
  Fcn/1 -> Mux/1
  Fcn1/1 -> Mux/3
  Mux/1 -> Om_dash|b/1

== system HSV/6DOF (Euler Angles) Rotating Earth/Angular Movments/OM/p, q, r/Om|g ==
  note: u1 = theta_dot, u2 = phi_dot, u3 = phi
  "theta_dot, phi_dot, phi" : Inport
  Fcn : Fcn  Expr=u(1)*cos(u(3))
  Fcn1 : Fcn  Expr=-u(1)*sin(u(3))
  Fcn2 : Fcn  Expr=-u(2)
  Mux : Mux  Inputs=3
  Om_dash|b : Outport
  wires:
  Mux/1 -> Om_dash|b/1
  Fcn1/1 -> Mux/3
  Fcn/1 -> Mux/1
  Fcn2/1 -> Mux/2
  "theta_dot, phi_dot, phi"/1 -> Fcn2/1, Fcn/1, Fcn1/1
